simulink subsystem "MEM"  (R2024b)
settings: Solver=VariableStepAuto  StartTime=0.0  StopTime=10.0  RelTol=1e-3
values from neighbouring files (symbols this model uses):
  modelStopCondition = "tohost"    [initSimuRISC.m]
  tohost_address = hex2dec('1000')    [initSimuRISC.m]
libraries: hdlsllib x9, simulink x3
settings Model: Creator=stefano  LastModifiedBy=stefano

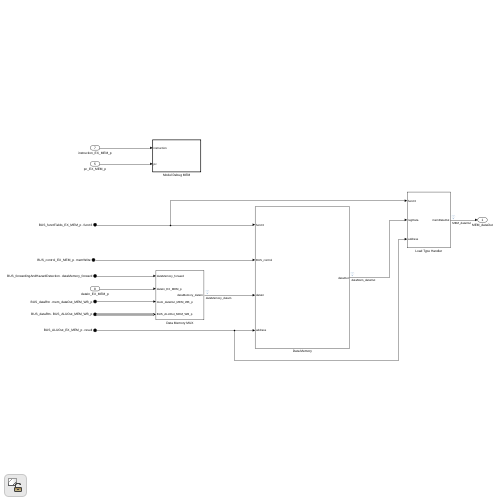
[thumbnail: Simulink's stored preview of the top-level diagram]
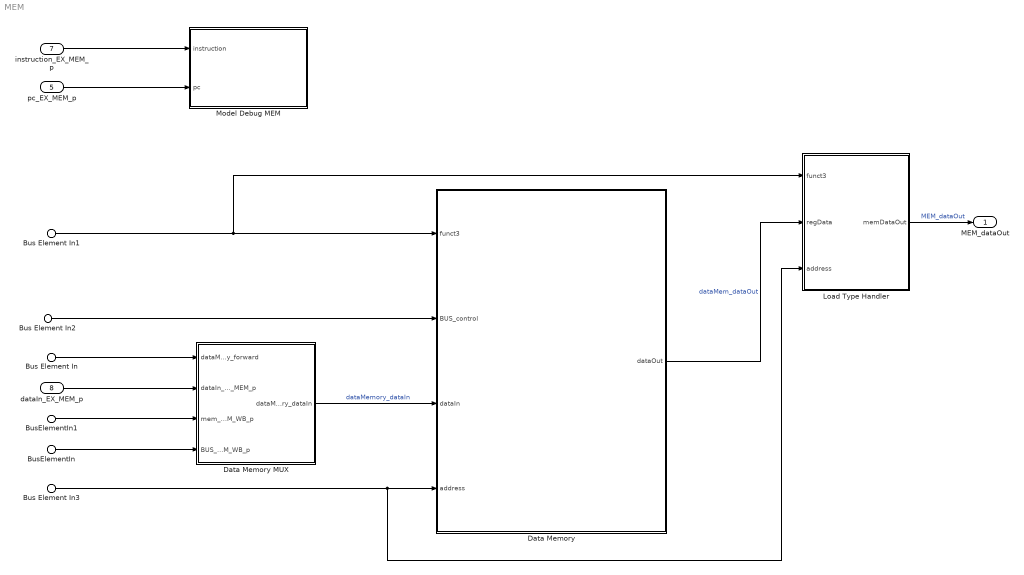
== system MEM ==
  BusElementIn : Inport  PortName=BUS_dataRtn  Element=BUS_ALUOut_MEM_WB_p
  BusElementIn1 : Inport  PortName=BUS_dataRtn  Element=mem_dataOut_MEM_WB_p
  Bus Element In : Inport  Port=2  PortName=BUS_forwardingAndHazardDetection  Element=dataMemory_forward
  Bus Element In1 : Inport  Port=3  PortName=BUS_functFields_EX_MEM_p  Element=funct3
  Bus Element In3 : Inport  Port=4  PortName=BUS_ALUOut_EX_MEM_p  Element=result
  pc_EX_MEM_p : Inport  Port=5
  Bus Element In2 : Inport  Port=6  PortName=BUS_control_EX_MEM_p  Element=memWrite
  instruction_EX_MEM_p : Inport  Port=7
  dataIn_EX_MEM_p : Inport  Port=8
  Data Memory : Subsystem
  Data Memory MUX : Subsystem
  Load Type Handler : Subsystem
  Model Debug MEM : Subsystem  TreatAsAtomicUnit=on
  MEM_dataOut : Outport
  wires:
  Data Memory/1(dataOut) -> Load Type Handler/2(regData)  "dataMem_dataOut"
  Bus Element In1/1 -> Data Memory/1(funct3), Load Type Handler/1(funct3)
  Data Memory MUX/1(dataMemory_dataIn) -> Data Memory/3(dataIn)  "dataMemory_dataIn"
  Bus Element In3/1 -> Data Memory/4(address), Load Type Handler/3(address)
  pc_EX_MEM_p/1 -> Model Debug MEM/2(pc)
  instruction_EX_MEM_p/1 -> Model Debug MEM/1(instruction)
  Load Type Handler/1(memDataOut) -> MEM_dataOut/1  "MEM_dataOut"
  Bus Element In2/1 -> Data Memory/2(BUS_control)
  BusElementIn1/1 -> Data Memory MUX/3(mem_dataOut_MEM_WB_p)
  dataIn_EX_MEM_p/1 -> Data Memory MUX/2(dataIn_EX_MEM_p)
  BusElementIn/1 -> Data Memory MUX/4(BUS_ALUOut_MEM_WB_p)
  Bus Element In/1 -> Data Memory MUX/1(dataMemory_forward)

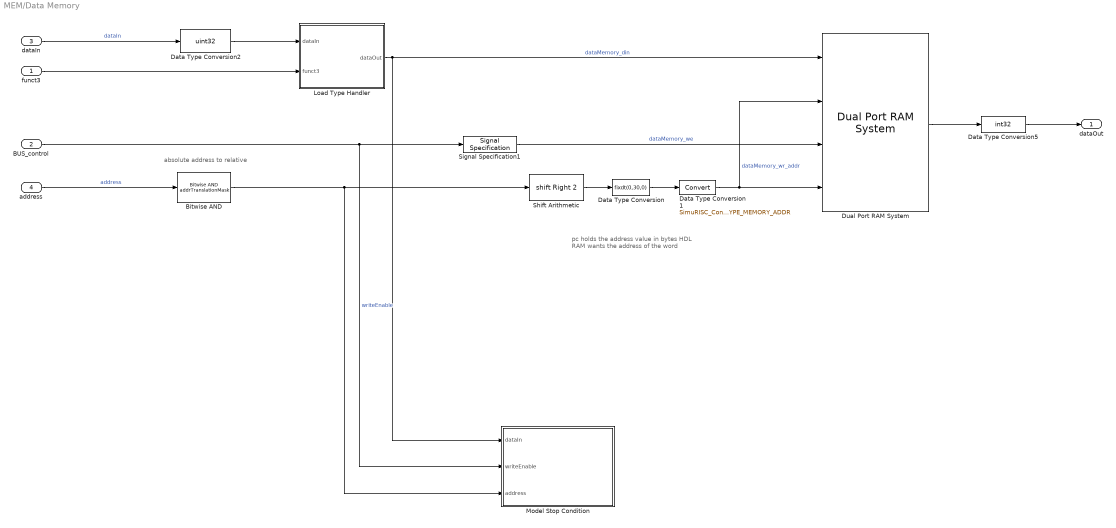
== system MEM/Data Memory ==
  note: absolute address to relative
  note: pc holds the address value in bytes
      | HDL RAM wants the address of the word
  funct3 : Inport
  BUS_control : Inport  Port=2
  dataIn : Inport  Port=3
  address : Inport  Port=4
  Bitwise AND : simulink/Logic and Bit Operations/Bitwise Operator  logicop=AND  UseBitMask=on  BitMask=addrTranslationMask  BitMaskRealWorld=Stored Integer
      settings: LibrarySourceBlock=|
      | simulink/Quick Insert/Logic and Bit
      | Operations/Bitwise AND
  Data Type Conversion : DataTypeConversion  OutDataTypeStr=fixdt(0,30,0)  SaturateOnIntegerOverflow=off  RndMeth=Floor
  Data Type Conversion1 : DataTypeConversion  OutDataTypeStr=SimuRISC_Constants.DATATYPE_MEMORY_ADDR  SaturateOnIntegerOverflow=off  RndMeth=Floor
  Data Type Conversion2 : DataTypeConversion  OutDataTypeStr=uint32  ConvertRealWorld=Stored Integer (SI)  SaturateOnIntegerOverflow=off  RndMeth=Floor
  Data Type Conversion5 : DataTypeConversion  OutDataTypeStr=int32  SaturateOnIntegerOverflow=off  RndMeth=Floor
  Dual Port RAM System : hdlsllib/HDL RAMs/Dual Port RAM System  RAMType=Simple dual port  AsyncRead=off  WriteOutputValue=New data  RAMInitialValue=dataMemory  allowBusInputs=off  WritesHaveOutput=on  NumReads=0  NumWrites=1  SimulateUsing=Code generation  ModelRAMDelay=off
  Load Type Handler : Subsystem
  Model Stop Condition : Subsystem  Variant=on  VariantControl=Subsystem  AllowZeroVariantControls=on
  Shift Arithmetic : ArithShift  BitShiftNumber=2  BitShiftDirection=Right
  Signal Specification1 : SignalSpecification  OutDataTypeStr=boolean
  dataOut : Outport
  wires:
  address/1 -> Bitwise AND/1  "address"
  BUS_control/1 -> Signal Specification1/1, Model Stop Condition/2(writeEnable)  "writeEnable"
  funct3/1 -> Load Type Handler/2(funct3)
  Bitwise AND/1 -> Model Stop Condition/3(address), Shift Arithmetic/1
  Data Type Conversion2/1 -> Load Type Handler/1(dataIn)
  Data Type Conversion5/1 -> dataOut/1
  Load Type Handler/1(dataOut) -> Dual Port RAM System/1, Model Stop Condition/1(dataIn)  "dataMemory_din"
  Signal Specification1/1 -> Dual Port RAM System/3  "dataMemory_we"
  Shift Arithmetic/1 -> Data Type Conversion/1
  Data Type Conversion1/1 -> Dual Port RAM System/4, Dual Port RAM System/2  "dataMemory_wr_addr"
  Dual Port RAM System/1 -> Data Type Conversion5/1
  dataIn/1 -> Data Type Conversion2/1  "dataIn"
  Data Type Conversion/1 -> Data Type Conversion1/1

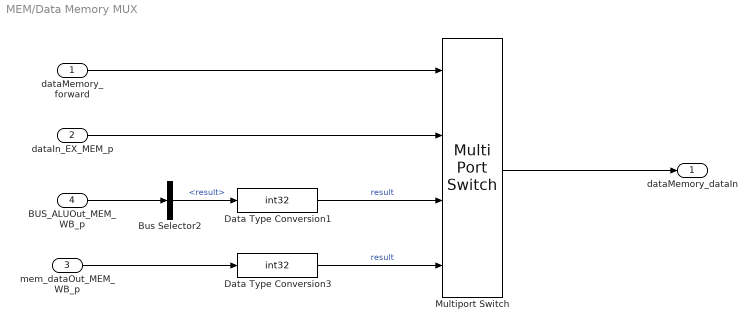
== system MEM/Data Memory MUX ==
  dataMemory_forward : Inport
  dataIn_EX_MEM_p : Inport  Port=2
  mem_dataOut_MEM_WB_p : Inport  Port=3
  BUS_ALUOut_MEM_WB_p : Inport  Port=4
  Bus Selector2 : BusSelector  OutputSignals=result
  Data Type Conversion1 : DataTypeConversion  OutDataTypeStr=int32  ConvertRealWorld=Stored Integer (SI)  SaturateOnIntegerOverflow=off  RndMeth=Floor
  Data Type Conversion3 : DataTypeConversion  OutDataTypeStr=int32  ConvertRealWorld=Stored Integer (SI)  SaturateOnIntegerOverflow=off  RndMeth=Floor
  Multiport Switch : MultiPortSwitch  DataPortOrder=Zero-based contiguous  zeroidx=on  SaturateOnIntegerOverflow=off  InputSameDT=off
  dataMemory_dataIn : Outport
  wires:
  Multiport Switch/1 -> dataMemory_dataIn/1
  Bus Selector2/1 -> Data Type Conversion1/1  "<result>"
  Data Type Conversion1/1 -> Multiport Switch/3  "result"
  Data Type Conversion3/1 -> Multiport Switch/4  "result"
  BUS_ALUOut_MEM_WB_p/1 -> Bus Selector2/1
  mem_dataOut_MEM_WB_p/1 -> Data Type Conversion3/1
  dataMemory_forward/1 -> Multiport Switch/1
  dataIn_EX_MEM_p/1 -> Multiport Switch/2

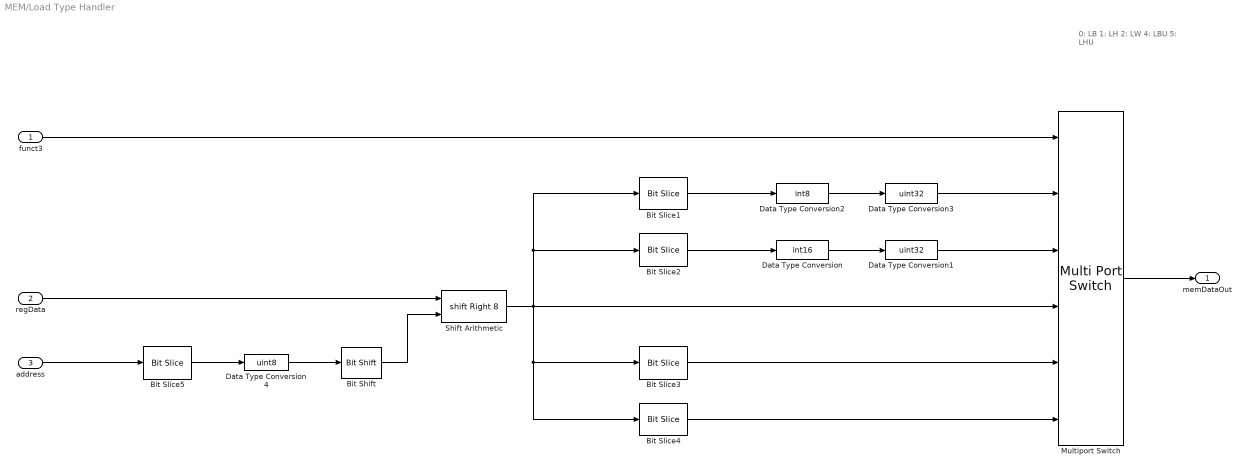
== system MEM/Load Type Handler ==
  note: 0: LB
      | 1: LH
      | 2: LW
      | 4: LBU
      | 5: LHU
  funct3 : Inport
  regData : Inport  Port=2
  address : Inport  Port=3
  Bit Shift : hdlsllib/Logic and Bit Operations/Bit Shift  mode=Shift Left Logical  N=3
  Bit Slice1 : hdlsllib/Logic and Bit Operations/Bit Slice  lidx=7  ridx=0
  Bit Slice2 : hdlsllib/Logic and Bit Operations/Bit Slice  lidx=15  ridx=0
  Bit Slice3 : hdlsllib/Logic and Bit Operations/Bit Slice  lidx=7  ridx=0
  Bit Slice4 : hdlsllib/Logic and Bit Operations/Bit Slice  lidx=15  ridx=0
  Bit Slice5 : hdlsllib/Logic and Bit Operations/Bit Slice  lidx=1  ridx=0
  Data Type Conversion : DataTypeConversion  OutDataTypeStr=int16  ConvertRealWorld=Stored Integer (SI)  SaturateOnIntegerOverflow=off  RndMeth=Floor
  Data Type Conversion1 : DataTypeConversion  OutDataTypeStr=uint32  ConvertRealWorld=Stored Integer (SI)  SaturateOnIntegerOverflow=off  RndMeth=Floor
  Data Type Conversion2 : DataTypeConversion  OutDataTypeStr=int8  ConvertRealWorld=Stored Integer (SI)  SaturateOnIntegerOverflow=off  RndMeth=Floor
  Data Type Conversion3 : DataTypeConversion  OutDataTypeStr=uint32  ConvertRealWorld=Stored Integer (SI)  SaturateOnIntegerOverflow=off  RndMeth=Floor
  Data Type Conversion4 : DataTypeConversion  OutDataTypeStr=uint8  SaturateOnIntegerOverflow=off  RndMeth=Floor
  Multiport Switch : MultiPortSwitch  DataPortOrder=Specify indices  Inputs=5  DataPortIndices={0,1,2,4,5}  DiagnosticForDefault=None  SaturateOnIntegerOverflow=off  InputSameDT=off
  Shift Arithmetic : ArithShift  BitShiftNumberSource=Input port  BitShiftNumber=8  BitShiftDirection=Right
      settings: InputPortMap=u0,p1
  memDataOut : Outport
  wires:
  address/1 -> Bit Slice5/1
  funct3/1 -> Multiport Switch/1
  Bit Slice3/1 -> Multiport Switch/5
  Data Type Conversion4/1 -> Bit Shift/1
  Bit Shift/1 -> Shift Arithmetic/2
  Bit Slice5/1 -> Data Type Conversion4/1
  regData/1 -> Shift Arithmetic/1
  Data Type Conversion2/1 -> Data Type Conversion3/1
  Data Type Conversion3/1 -> Multiport Switch/2
  Data Type Conversion1/1 -> Multiport Switch/3
  Data Type Conversion/1 -> Data Type Conversion1/1
  Bit Slice4/1 -> Multiport Switch/6
  Bit Slice1/1 -> Data Type Conversion2/1
  Shift Arithmetic/1 -> Multiport Switch/4, Bit Slice1/1, Bit Slice2/1, Bit Slice3/1, Bit Slice4/1
  Bit Slice2/1 -> Data Type Conversion/1
  Multiport Switch/1 -> memDataOut/1

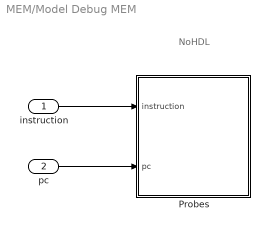
== system MEM/Model Debug MEM ==
  note: NoHDL
  instruction : Inport
  pc : Inport  Port=2
  Probes : Subsystem
  wires:
  pc/1 -> Probes/2(pc)
  instruction/1 -> Probes/1(instruction)

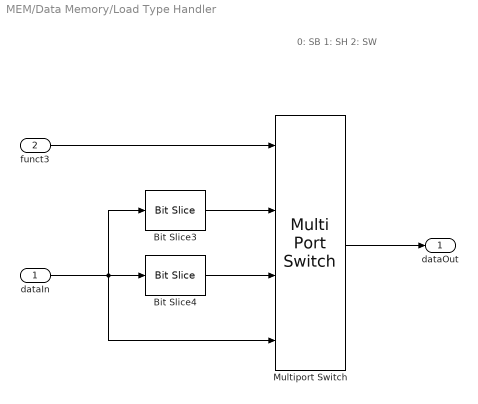
== system MEM/Data Memory/Load Type Handler ==
  note: 0: SB
      | 1: SH
      | 2: SW
  dataIn : Inport
  funct3 : Inport  Port=2
  Bit Slice3 : hdlsllib/Logic and Bit Operations/Bit Slice  lidx=7  ridx=0
  Bit Slice4 : hdlsllib/Logic and Bit Operations/Bit Slice  lidx=15  ridx=0
  Multiport Switch : MultiPortSwitch  DataPortOrder=Zero-based contiguous  DataPortIndices={0,1,2,4,5}  DiagnosticForDefault=None  zeroidx=on  SaturateOnIntegerOverflow=off  InputSameDT=off
  dataOut : Outport
  wires:
  funct3/1 -> Multiport Switch/1
  dataIn/1 -> Bit Slice4/1, Multiport Switch/4, Bit Slice3/1
  Bit Slice3/1 -> Multiport Switch/2
  Bit Slice4/1 -> Multiport Switch/3
  Multiport Switch/1 -> dataOut/1

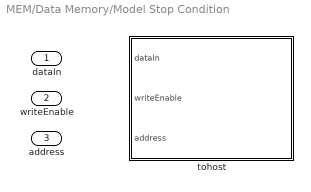
== system MEM/Data Memory/Model Stop Condition ==
  dataIn : Inport
  writeEnable : Inport  Port=2
  address : Inport  Port=3
  tohost : Subsystem  VariantControl="strcmp(modelStopCondition, \"tohost\")"

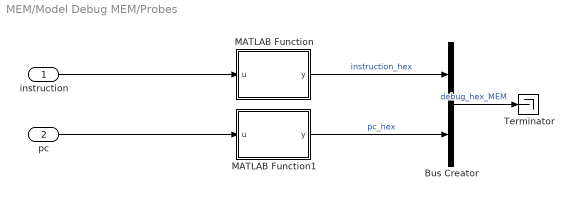
== system MEM/Model Debug MEM/Probes ==
  instruction : Inport
  pc : Inport  Port=2
  Bus Creator : BusCreator  Inputs=2
  MATLAB Function : MATLAB Function  TreatAsAtomicUnit=on
  MATLAB Function1 : MATLAB Function  TreatAsAtomicUnit=on
  Terminator : Terminator
  wires:
  MATLAB Function1/1(y) -> Bus Creator/2  "pc_hex"
  Bus Creator/1 -> Terminator/1  "debug_hex_MEM"
  instruction/1 -> MATLAB Function/1(u)
  pc/1 -> MATLAB Function1/1(u)
  MATLAB Function/1(y) -> Bus Creator/1  "instruction_hex"

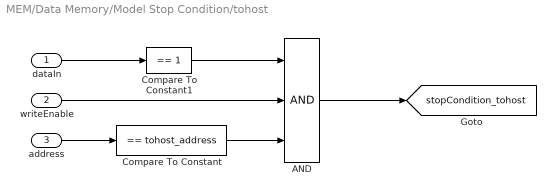
== system MEM/Data Memory/Model Stop Condition/tohost ==
  dataIn : Inport
  writeEnable : Inport  Port=2
  address : Inport  Port=3
  AND : Logic  Inputs=3  IconShape=distinctive  AllPortsSameDT=off  OutDataTypeStr=boolean
  Compare To Constant : simulink/Logic and Bit Operations/Compare To Constant  relop===  const=tohost_address  OutDataTypeStr=boolean
  Compare To Constant1 : simulink/Logic and Bit Operations/Compare To Constant  relop===  const=1  OutDataTypeStr=boolean
  tag scope: stopCondition_tohost=global
  wires:
  writeEnable/1 -> AND/2
  dataIn/1 -> Compare To Constant1/1
  AND/1 -> [stopCondition_tohost]
  address/1 -> Compare To Constant/1
  Compare To Constant1/1 -> AND/1
  Compare To Constant/1 -> AND/3

== matlab function MEM/Model Debug MEM/Probes/MATLAB Function1 ==
  data: u input; y output string
function y = toHex(u)

y = string(dec2hex(u, 8));

== matlab function MEM/Model Debug MEM/Probes/MATLAB Function ==
  data: u input; y output string
function y = toHex(u)

y = string(dec2hex(u, 8));
